simulink model "Node_N"  (R2024b)
settings: Solver=ode1  StartTime=0.0  StopTime=10.0  FixedStep=0.5e-3  RelTol=1e-3
settings Model: DataDictionary=N_dd.sldd  EnableAccessToBaseWorkspace=off  NumberOfSteps=1000  Creator=wai484  LastModifiedBy=wai484
settings SolverCC: EnableFixedStepZeroCrossing=on
settings DataIOCC: SaveOutput=off  SaveTime=off
settings OptimizationCC: UseDivisionForNetSlopeComputation=UseDivisionForReciprocalsOfIntegersOnly  StateBitsets=on  DataBitsets=on  EfficientFloat2IntCast=on  SimCompilerOptimization=on
settings DebuggingCC: SignalInfNanChecking=error  SignalRangeChecking=error  ReadBeforeWriteMsg=EnableAllAsError  WriteAfterWriteMsg=EnableAllAsError  WriteAfterReadMsg=EnableAllAsError  AlgebraicLoopMsg=error  ArtificialAlgebraicLoopMsg=error  SaveWithDisabledLinksMsg=error  SaveWithParameterizedLinksMsg=error  BlockPriorityViolationMsg=error  SolverPrmCheckMsg=error  InheritedTsInSrcMsg=error  TasksWithSamePriorityMsg=error  SigSpecEnsureSampleTimeMsg=error  CheckMatrixSingularityMsg=error  IntegerOverflowMsg=error  ParameterUnderflowMsg=error  ParameterPrecisionLossMsg=error  ParameterTunabilityLossMsg=error  UnderSpecifiedDataTypeMsg=error  UnnecessaryDatatypeConvMsg=warning  VectorMatrixConversionMsg=error  UnconnectedInputMsg=error  UnconnectedOutputMsg=error  UnconnectedLineMsg=error  SFcnCompatibilityMsg=error  UniqueDataStoreMsg=error  BusObjectLabelMismatch=error  RootOutportRequireBusObject=error  AssertControl=DisableAll  ModelReferenceIOMismatchMessage=error  UnknownTsInhSupMsg=error  ModelReferenceDataLoggingMessage=error  StateNameClashWarn=warning  StrictBusMsg=ErrorOnBusTreatedAsVector  NonBusSignalsTreatedAsBus=error  SFInvalidInputDataAccessInChartInitDiag=error  SFTransitionOutsideNaturalParentDiag=error  SFUnreachableExecutionPathDiag=error  SFUndirectedBroadcastEventsDiag=error  SFTransitionActionBeforeConditionDiag=error  SFTemporalDelaySmallerThanSampleTimeDiag=error  SFSelfTransitionDiag=error  SFExecutionAtInitializationDiag=error  IntegerSaturationMsg=error  VariantConditionMismatch=error
settings ModelReferenceCC: EnableParallelModelReferenceBuilds=on
settings SFSimCC: CompileTimeRecursionLimit=0  EnableRuntimeRecursion=off  MATLABDynamicMemAlloc=off  SimHardwareAcceleration=native
settings RTWCC: BuildConfiguration=Faster Runs
settings GRTTargetCC: UtilityFuncGeneration=Shared location  CombineOutputUpdateFcns=off  MatFileLogging=off  SupportNonFinite=off  OptimizeReductions=on

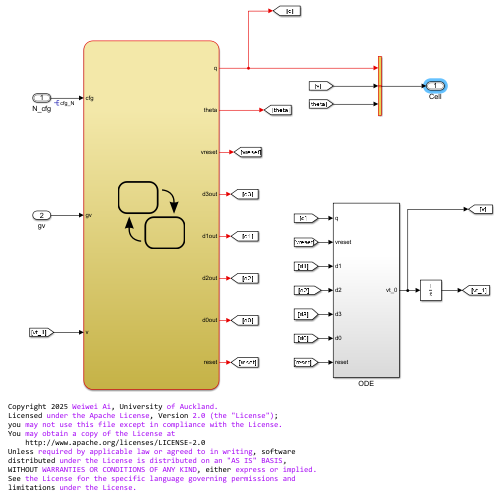
[thumbnail: Simulink's stored preview of the top-level diagram]
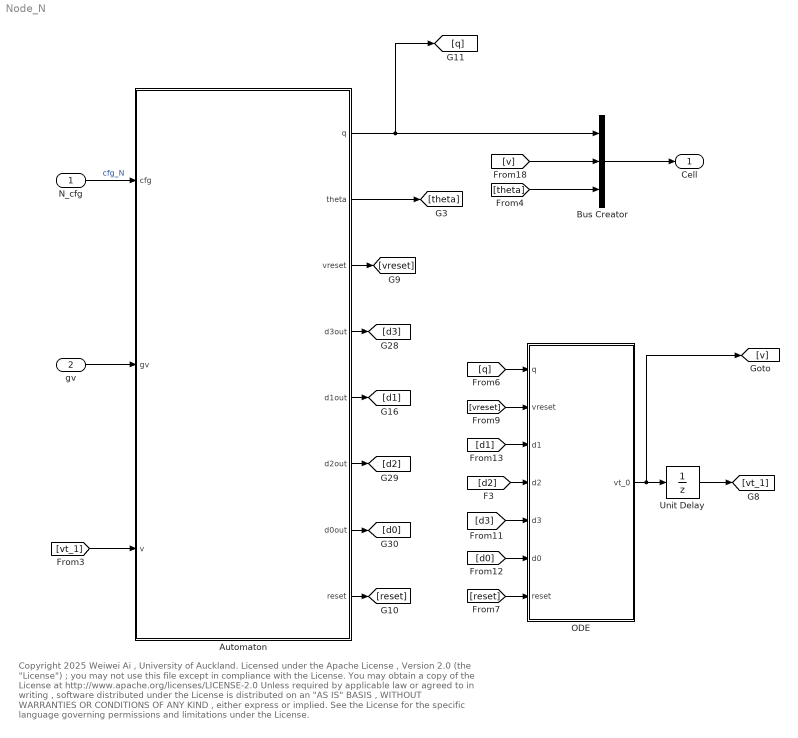
== system Node_N ==
  note: Copyright 2025 Weiwei Ai , University of Auckland.
      | Licensed under the Apache License , Version 2.0 (the "License") ;
      | you may not use this file except in compliance with the License.
      | You may obtain a copy of the License at
      | http://www.apache.org/licenses/LICENSE-2.0
      | Unless required by applicable law or agreed to in writing , software
      | distributed under the License is distributed on an "AS IS" BASIS ,
      | WITHOUT WARRANTIES OR CONDITIONS OF ANY KIND , either express or implied.
      | See the License for the specific language governing permissions and
      | limitations under the License.
  N_cfg : Inport  OutDataTypeStr=Bus: Config_N  BusOutputAsStruct=on
  gv : Inport  Port=2  OutDataTypeStr=double  PortDimensions=1
  Automaton : Stateflow chart  TreatAsAtomicUnit=on
  Bus Creator : BusCreator  Inputs=3  OutDataTypeStr=Bus: Cell  NonVirtualBus=on
      settings: InheritFromInputs=off
  ODE : Subsystem
  Unit Delay : UnitDelay  SampleTime=-1  HasFrameUpgradeWarning=on
  Cell : Outport  OutDataTypeStr=Bus: Cell  BusOutputAsStruct=on
  wires:
  Automaton/1(q) -> Bus Creator/1, [q]
  [d1] -> ODE/3(d1)
  [d2] -> ODE/4(d2)
  [d3] -> ODE/5(d3)
  [d0] -> ODE/6(d0)
  Automaton/3(vreset) -> [vreset]
  Automaton/8(reset) -> [reset]
  [q] -> ODE/1(q)
  [reset] -> ODE/7(reset)
  [vreset] -> ODE/2(vreset)
  [v] -> Bus Creator/2
  [theta] -> Bus Creator/3
  Automaton/2(theta) -> [theta]
  Automaton/5(d1out) -> [d1]
  Automaton/4(d3out) -> [d3]
  Automaton/6(d2out) -> [d2]
  Automaton/7(d0out) -> [d0]
  [vt_1] -> Automaton/3(v)
  N_cfg/1 -> Automaton/1(cfg)  "cfg_N"
  ODE/1(vt_0) -> [v], Unit Delay/1
  Unit Delay/1 -> [vt_1]
  gv/1 -> Automaton/2(gv)
  Bus Creator/1 -> Cell/1

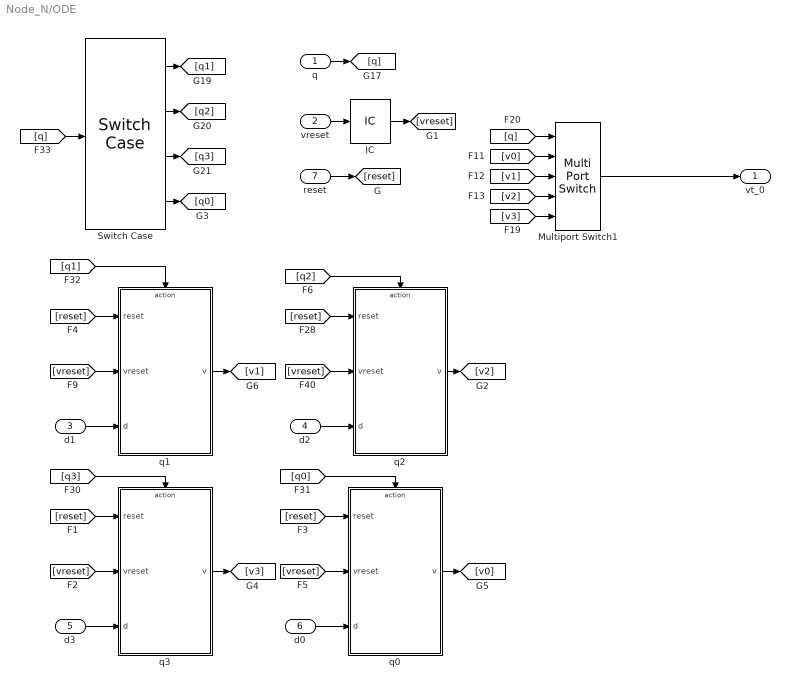
== system Node_N/ODE ==
  q : Inport
  vreset : Inport  Port=2
  d1 : Inport  Port=3
  d2 : Inport  Port=4
  d3 : Inport  Port=5
  d0 : Inport  Port=6
  reset : Inport  Port=7
  IC : InitialCondition  Value=0
  Multiport Switch1 : MultiPortSwitch  DataPortOrder=Zero-based contiguous  Inputs=4  zeroidx=on  SaturateOnIntegerOverflow=off  InputSameDT=off
  Switch Case : SwitchCase  CaseConditions={1,2,3,0}  ShowDefaultCase=off
  q0 : Subsystem  TreatAsAtomicUnit=on
  q1 : Subsystem  TreatAsAtomicUnit=on
  q2 : Subsystem  TreatAsAtomicUnit=on
  q3 : Subsystem  TreatAsAtomicUnit=on
  vt_0 : Outport
  wires:
  d1/1 -> q1/3(d)
  [vreset] -> q1/2(vreset)
  [reset] -> q2/1(reset)
  [v3] -> Multiport Switch1/5
  [v2] -> Multiport Switch1/4
  [v1] -> Multiport Switch1/3
  [v0] -> Multiport Switch1/2
  Multiport Switch1/1 -> vt_0/1
  [q0] -> q0/Action
  [q3] -> q3/Action
  [vreset] -> q0/2(vreset)
  [reset] -> q0/1(reset)
  d0/1 -> q0/3(d)
  q0/1(v) -> [v0]
  [vreset] -> q3/2(vreset)
  [reset] -> q3/1(reset)
  d3/1 -> q3/3(d)
  q3/1(v) -> [v3]
  [vreset] -> q2/2(vreset)
  [q2] -> q2/Action
  d2/1 -> q2/3(d)
  q2/1(v) -> [v2]
  Switch Case/4 -> [q0]
  Switch Case/3 -> [q3]
  Switch Case/2 -> [q2]
  Switch Case/1 -> [q1]
  [reset] -> q1/1(reset)
  [q1] -> q1/Action
  [q] -> Switch Case/1
  [q] -> Multiport Switch1/1
  q1/1(v) -> [v1]
  q/1 -> [q]
  reset/1 -> [reset]
  vreset/1 -> IC/1
  IC/1 -> [vreset]

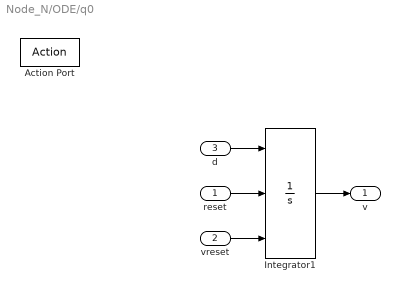
== system Node_N/ODE/q0 ==
  reset : Inport
  vreset : Inport  Port=2
  d : Inport  Port=3
  Action Port : ActionPort  InitializeStates=reset  ActionPortLabel=case [ 0 ]:
  Integrator1 : Integrator  ExternalReset=either  InitialConditionSource=external  InitialCondition=20
  v : Outport
  wires:
  Integrator1/1 -> v/1
  reset/1 -> Integrator1/2
  vreset/1 -> Integrator1/3
  d/1 -> Integrator1/1

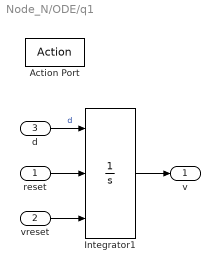
== system Node_N/ODE/q1 ==
  reset : Inport
  vreset : Inport  Port=2
  d : Inport  Port=3
  Action Port : ActionPort  InitializeStates=reset  ActionPortLabel=case [ 1 ]:
  Integrator1 : Integrator  ExternalReset=either  InitialConditionSource=external  InitialCondition=20
  v : Outport
  wires:
  d/1 -> Integrator1/1  "d"
  Integrator1/1 -> v/1
  reset/1 -> Integrator1/2
  vreset/1 -> Integrator1/3

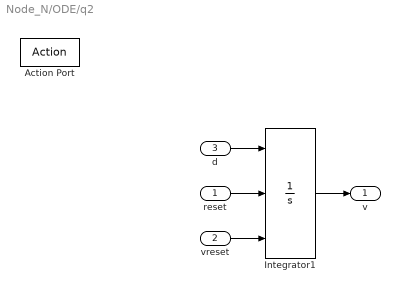
== system Node_N/ODE/q2 ==
  reset : Inport
  vreset : Inport  Port=2
  d : Inport  Port=3
  Action Port : ActionPort  InitializeStates=reset  ActionPortLabel=case [ 2 ]:
  Integrator1 : Integrator  ExternalReset=either  InitialConditionSource=external  InitialCondition=20
  v : Outport
  wires:
  d/1 -> Integrator1/1
  vreset/1 -> Integrator1/3
  reset/1 -> Integrator1/2
  Integrator1/1 -> v/1

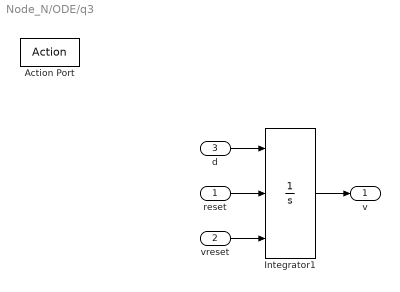
== system Node_N/ODE/q3 ==
  reset : Inport
  vreset : Inport  Port=2
  d : Inport  Port=3
  Action Port : ActionPort  InitializeStates=reset  ActionPortLabel=case [ 3 ]:
  Integrator1 : Integrator  ExternalReset=either  InitialConditionSource=external  InitialCondition=20
  v : Outport
  wires:
  Integrator1/1 -> v/1
  reset/1 -> Integrator1/2
  vreset/1 -> Integrator1/3
  d/1 -> Integrator1/1

== stateflow chart Node_N/Automaton ==
  settings: updateMethod=DISCRETE
  state PacemakerCell
    state Cell [parallel]
      settings: executionOrder=1
      state Slow
        en: q=1; %phase4
      state Stimulated
        en: q=2; %phase0
        f1theta=exp(-h*theta);
        Vmax=(-1)*MDP*f1theta;
        [f3theta,n,Vmin]=sat(n,hr,hs,Vh1,s,m,theta);
      state Plateau
        en: q=3;%phase2
      state RP
        en:q=0;%phase3
      (default) -> Slow : /{Vmin=0;Vmax=(-1)*MDP; d3=d3fcn(MDP,VR,VT,d0,d2,ERP); BCL=RR(cfg_default_N,t);...
          | t3=(abs(MDP)-VR)/abs(d3); t0=VR/abs(d0);t2=(abs(MDP)-VT)/abs(d2);d1=(VT)/(BCL-t3-t0-t2);d1out=d1;}
      Slow -> Stimulated [order 1] : [gv>VT&& v<VT]{theta=(v-VT)/(Vmin-VT);f2theta=exp(-f*theta);d2out=d2*f2theta;...
          |  f4theta=exp(j*(theta-1)); Vh1=Vh*f4theta; n=n+1;  ...
          |  vreset=v;reset; }
      Slow -> Stimulated [order 2] : [v>=VT]{theta=0; f2theta=exp(-f*theta); d2out=d2*f2theta;...
          |  n=(1-r)*n;  vreset=v;reset; }
      RP -> Slow : [v<=Vmin]{t3=(abs(MDP)-VR)/abs(d3); t0=VR/abs(d0);...
          | t2=(abs(MDP)-VT)/abs(d2);
          | BCL=RR(cfg,t);
          | d1=(VT)/(BCL-t3-t0-t2); d1out=d1*f3theta;...
          | [d2,ERP,d0,MDP,VT,VR,Vh,hr,hs,s,j,m,h,f,r]=get_cfg(cfg);
          | vreset=v;reset;}
      Stimulated -> Plateau : [v>=Vmax]{d3=d3fcn(MDP,VR,VT,d0,d2,ERP);...
          | d3out=d3*f2theta;...
          | vreset=v;reset;}
      Plateau -> RP : [v<=VR]{d0out=d0*f2theta; vreset=v;reset;}
    state R [parallel]
      du:
      t=temporalCount(sec);
      settings: executionOrder=2
  (default) -> PacemakerCell : {t=0; [d2,ERP,d0,MDP,VT,VR,Vh,hr,hs,s,j,m,h,f,r]=get_cfg(cfg_default_N);}
  data: pcfg function_input Bus: Config_N; pd2 function_output double; pERP function_output double; pd0 function_output double; pMDP function_output double; pVT function_output double; pVR function_output double; pVh function_output double; phr function_output double; phs function_output double; ps function_output double; pj function_output double; pm function_output double; ph function_output double; pf function_output double; pr function_output double; f3out function_output double; tout function_output double; pt function_input double; Vminout function_output double; phr function_input double; phs function_input double; pVh function_input double; ps function_input double; pm function_input double; ptheta function_input double; pMDP function_input double; pVR function_input double; pVT function_input double; pd0 function_input double; pd2 function_input double; pERP function_input double; d3in function_output double; pcfg function_input Bus: Config_N; rr function_output double size=1; pt function_input double; q output int8; cfg input Bus: Config_N =0; Vmax local double; theta output double; vreset output double =0; gv input; v input double; f1theta local double; Vh1 local double; Vmin local double; d3out output double; d1out output double; Vtemp local double; t local double; f3theta local double; d2out output double; d0out output double; f2theta local double; n local double; f4theta local double; d2 local double; Vh local double; h local double; hr local double; hs local double; j local double; m local double; r local double; s local double; BCL local double; ERP local double; MDP local double; VR local double; VT local double; d0 local double; f local double; d1 local double; d3 local double; t0 local double; t2 local double; t3 local double; cfg_default_N parameter Bus: Config_N
  data v settings: updateMethod=SF_CONTINUOUS_TIME_DATA
  events: reset output EITHER_EDGE_EVENT
  function [pd2,pERP,pd0,pMDP,pVT,pVR,pVh,phr,phs,ps,pj,pm,ph,pf,pr]=get_cfg(pcfg):
    | function [pd2,pERP,pd0,pMDP,pVT,pVR,pVh,phr,phs,ps,pj,pm,ph,pf,pr]=get_cfg(pcfg)
    | %#codegen
    | pd2=pcfg.d2;
    | pERP=pcfg.ERP;
    | pd0=pcfg.d0;
    | pMDP=pcfg.MDP;
    | pVT=pcfg.VT;
    | pVR=pcfg.VR;
    | pVh=pcfg.Vh;
    | phr=pcfg.hr;
    | phs=pcfg.hs;
    | ps=pcfg.s;
    | pj=pcfg.j;
    | pm=pcfg.m;
    | ph=pcfg.h;
    | pf=pcfg.f;
    | pr=pcfg.r;
  function [f3out,tout,Vminout]=sat(pt,phr,phs,pVh,ps,pm,ptheta):
    | function [f3out,tout,Vminout]=sat(pt,phr,phs,pVh,ps,pm,ptheta)
    | 
    | td=phr*(pt-phs);
    | 
    | if td>=5
    |     tout=5/phr+phs;
    | else
    |     tout=pt;
    | end
    | 
    | if tout<1
    | co=0;
    | else
    | Vtemp=1+exp(-phr*(tout-phs)); 
    | co=1/Vtemp;
    | end
    | Vminout=pVh*co;
    | thetai=ptheta;
    | for i=1:ps-1
    |     thetai=thetai*ptheta;
    | end
    | ft=pm*co*thetai+1;
    | f3out=1/ft;
    | end
  function d3in= d3fcn(pMDP,pVR,pVT,pd0,pd2,pERP):
    | function d3in= d3fcn(pMDP,pVR,pVT,pd0,pd2,pERP)
    | %#codegen
    | d3in=-(abs(pMDP)-pVR)/(pERP-(abs(pMDP)-pVT)/pd2-pVR/abs(pd0));
  function rr= RR(pcfg,pt):
    | function rr= RR(pcfg,pt)
    | %Rate dependent factor
    | c1=0.01;
    | c2=0.01;
    | if pcfg.sigma1sq<0 || pcfg.sigma2sq<0
    |     error('Invalid input');
    | end
    | % The Gaussian frequency distribution, power spectrum
    | hf=0.5;
    | fstep=0.025;
    | ff=0:fstep:hf; % The frequency range original;
    | % fmax=1; % Assume the highest frequency
    | % fmin=0.025; % Assume the lowest frequency
    | % Fs=2*fmax; % The sample frequency 
    | % tstep=1/Fs; % The sample period of the time series
    | % tmax=1/fmin; % The period of the time series
    | % N=tmax/tstep;
    | % fstep=2*fmax/N; % =fmin
    | % f=fstep:fstep:fmax; % The frequency range original; 
    | ln=length(ff); % The number of frequency/cos signals.
    | s1=(pcfg.sigma1sq/(c1*sqrt(2*pi)))*exp(-(ff-pcfg.f1).^2/(2*c1^2));
    | s2=(pcfg.sigma2sq/(c2*sqrt(2*pi)))*exp(-(ff-pcfg.f2).^2/(2*c2^2));
    | ss=s1+s2; % s(f)
    | rss=sqrt(ss); %
    | %Construct the time series y(t) from s(f);
    | mag=rss; % the amplitudes;
    | y = ff'*2*pi*pt;
    | y = cos(y);
    | for i=1:ln
    |     y(i,:)=y(i,:)*mag(i);
    | end
    | if ln>1
    |     y1=sum(y);
    | else
    |     y1=y;
    | end
    | rr=pcfg.BCL+y1*pcfg.SD;
    | end
